simulink model "CPA1_1"  (R2012b)
settings: Solver=ode1  StartTime=0.0  StopTime=3  FixedStep=0.05  RelTol=1e-3
libraries: opclib x5
settings Model: Creator=Leonardo  LastModifiedBy=Josias
settings DataIOCC: SignalLoggingSaveFormat=ModelDataLogs
settings OptimizationCC: ExpressionDepthLimit=128
settings DebuggingCC: UnderspecifiedInitializationDetection=Simplified  MultiTaskDSMMsg=warning  MultiTaskCondExecSysMsg=none  StateNameClashWarn=none  StrictBusMsg=None
settings RTWCC: IncludeERTFirstTime=on
settings CodeAppCC: CustomSymbolStrType=$N$R$M_T  InternalIdentifier=Shortened
settings GRTTargetCC: CodeReplacementLibrary=None  CPPClassGenCompliant=on

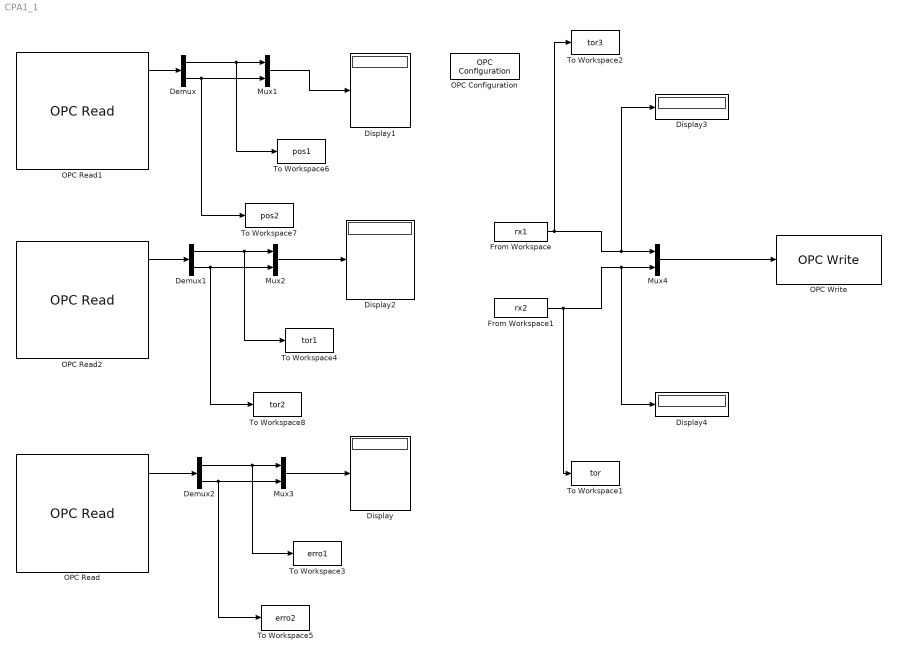
== system CPA1_1 ==
  Demux : Demux  Outputs=2
  Demux1 : Demux  Outputs=2
  Demux2 : Demux  Outputs=2
  Display{,1..4} (5 alike) : Display
  From Workspace : FromWorkspace  VariableName=rx1  SampleTime=0
  From Workspace1 : FromWorkspace  VariableName=rx2  SampleTime=0
  Mux{1..4} (4 alike) : Mux  Inputs=2
  OPC Configuration : opclib/OPC Configuration  opcServers=localhost/ElipseSCADA.OPCSvr.1/10  errMissingItems=Error  errReadWrite=Warn  errShutdown=Error  errRTViolation=Warn  rtEnable=on  speedup=1  showLatency=off  beingUsed=on
  OPC Read : opclib/OPC Read  serverHost=localhost  serverID=ElipseSCADA.OPCSvr.1  itemIDs=Tags.Erro_J1, Tags.Erro_J2  readMode=Synchronous (cache)  dataType=double  updateRate=0.05  showQual=on  showTS=on  tsMode=Seconds since start
  OPC Read1 : opclib/OPC Read  serverHost=localhost  serverID=ElipseSCADA.OPCSvr.1  itemIDs=Tags.posição1, Tags.Posição2  readMode=Synchronous (cache)  dataType=double  updateRate=0.05  showQual=on  showTS=on  tsMode=Seconds since start
  OPC Read2 : opclib/OPC Read  serverHost=localhost  serverID=ElipseSCADA.OPCSvr.1  itemIDs=Tags.sinal_junta_1, Tags.sinal_junta_2  readMode=Synchronous (cache)  dataType=double  updateRate=0.05  showQual=on  showTS=on  tsMode=Seconds since start
  OPC Write : opclib/OPC Write  serverHost=localhost  serverID=ElipseSCADA.OPCSvr.1  itemIDs=Tags.setpoint_teta_1, Tags.setpoint_teta_2  writeMode=Synchronous  updateRate=0.05
  To Workspace1 : ToWorkspace  VariableName=tor  SampleTime=-1
  To Workspace2 : ToWorkspace  VariableName=tor3  SampleTime=-1
  To Workspace3 : ToWorkspace  VariableName=erro1  SampleTime=-1
  To Workspace4 : ToWorkspace  VariableName=tor1  SampleTime=-1
  To Workspace5 : ToWorkspace  VariableName=erro2  SampleTime=-1
  To Workspace6 : ToWorkspace  VariableName=pos1  SampleTime=-1
  To Workspace7 : ToWorkspace  VariableName=pos2  SampleTime=-1
  To Workspace8 : ToWorkspace  VariableName=tor2  SampleTime=-1
  wires:
  Demux/2 -> To Workspace7/1, Mux1/2
  Demux/1 -> To Workspace6/1, Mux1/1
  OPC Read1/1 -> Demux/1
  Demux1/2 -> To Workspace8/1, Mux2/2
  Demux1/1 -> To Workspace4/1, Mux2/1
  OPC Read2/1 -> Demux1/1
  Mux2/1 -> Display2/1
  Demux2/2 -> To Workspace5/1, Mux3/2
  Demux2/1 -> To Workspace3/1, Mux3/1
  OPC Read/1 -> Demux2/1
  Mux3/1 -> Display/1
  Mux1/1 -> Display1/1
  Mux4/1 -> OPC Write/1
  From Workspace/1 -> To Workspace2/1, Display3/1, Mux4/1
  From Workspace1/1 -> To Workspace1/1, Display4/1, Mux4/2
